simulink model "Ue6_Aufgabe2a"  (R2017a)
settings: Solver=VariableStepAuto  StartTime=0.0  StopTime=50000  RelTol=1e-3
undefined symbols (not defined in the file or in its folder): entity, m, n, showValue, timeStamp
settings Model: Creator=gome  LastModifiedBy=gome

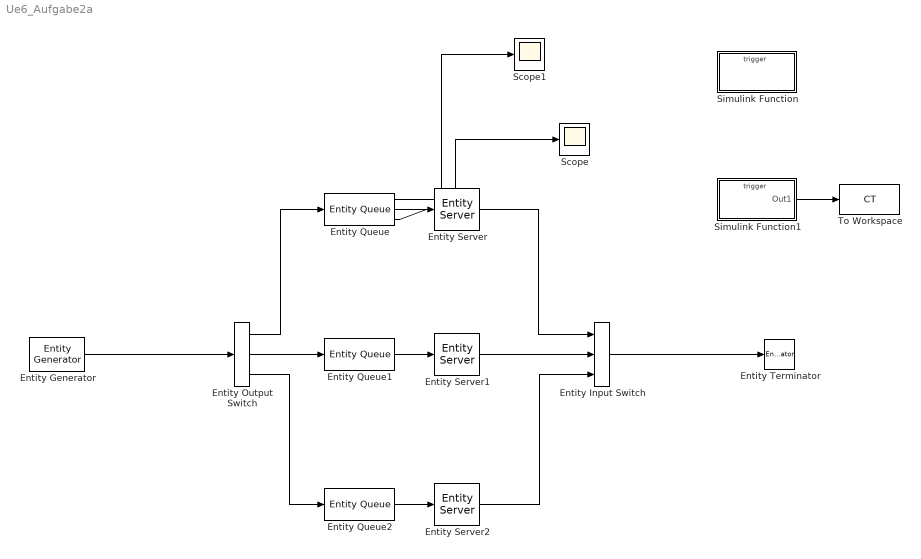
== system Ue6_Aufgabe2a ==
  Entity Input Switch : EntityInputSwitch  InputPortMessageModes=m,m,m  OutputPortMessageModes=m  NumberInputPorts=3
      settings: InputPortMap=u1,u2,u3
  Entity Output Switch : EntityOutputSwitch  InputPortMessageModes=m  OutputPortMessageModes=m,m,m  NumberOutputPorts=3  SwitchingCriterion=Equiprobable  SwitchAttributeName=Attribute1
      settings: OutputPortMap=o0,o1,o2
  Entity Generator : EntityGenerator  OutputPortMessageModes=m  TimeSource=MATLAB action  IntergenerationTimeAction=|  GenerateAction=entity.startTime = timeStamp();  AttributeName=startTime  EntityType=Structured  EntityTypeName=Entity
      | persistent init
      | if isempty(init)
      |     init = 1;
      |     rng(75241);
      | end
      | dt = exprnd(1/2);
  Entity Queue : EntityQueue  InputPortMessageModes=m  OutputPortMessageModes=n,n,m  Capacity=inf  AverageWait=on  AverageQueueLength=on
      settings: OutputPortMap=o2,o3,o5
  Entity Queue1 : EntityQueue  InputPortMessageModes=m  OutputPortMessageModes=m  Capacity=inf
      settings: OutputPortMap=o5
  Entity Queue2 : EntityQueue  InputPortMessageModes=m  OutputPortMessageModes=m  Capacity=inf
      settings: OutputPortMap=o5
  Entity Server : EntityServer  InputPortMessageModes=m  OutputPortMessageModes=m  Capacity=1  ServiceTimeSource=MATLAB action  ServiceTimeAction=|
      | persistent init
      | if isempty(init)
      |     init = 1;
      |     rng(945);
      | end
      | dt = exprnd(1);
  Entity Server1 : EntityServer  InputPortMessageModes=m  OutputPortMessageModes=m  Capacity=1  ServiceTimeSource=MATLAB action  ServiceTimeAction=|
      | persistent init
      | if isempty(init)
      |     init = 1;
      |     rng(1323456);
      | end
      | dt = exprnd(1);
  Entity Server2 : EntityServer  InputPortMessageModes=m  OutputPortMessageModes=m  Capacity=1  ServiceTimeSource=MATLAB action  ServiceTimeAction=|
      | persistent init
      | if isempty(init)
      |     init = 1;
      |     rng(52434);
      | end
      | dt = 0.5+1.5*rand;
  Entity Terminator : EntityTerminator  InputPortMessageModes=m  EntryAction=showValue(timeStamp-entity.startTime);
  Scope : Scope
  Scope1 : Scope
  Simulink Function : Subsystem  TreatAsAtomicUnit=on
  Simulink Function1 : Subsystem  TreatAsAtomicUnit=on
  To Workspace : ToWorkspace  VariableName=CT  SampleTime=-1
  wires:
  Entity Generator/1 -> Entity Output Switch/1
  Entity Output Switch/1 -> Entity Queue/1
  Entity Output Switch/2 -> Entity Queue1/1
  Entity Output Switch/3 -> Entity Queue2/1
  Entity Queue/3 -> Entity Server/1
  Entity Queue1/1 -> Entity Server1/1
  Entity Queue2/1 -> Entity Server2/1
  Entity Server/1 -> Entity Input Switch/1
  Entity Server1/1 -> Entity Input Switch/2
  Entity Server2/1 -> Entity Input Switch/3
  Entity Input Switch/1 -> Entity Terminator/1
  Simulink Function1/1(Out1) -> To Workspace/1
  Entity Queue/1 -> Scope/1
  Entity Queue/2 -> Scope1/1

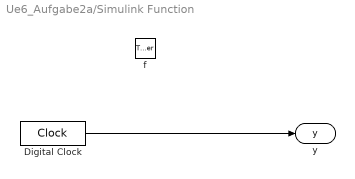
== system Ue6_Aufgabe2a/Simulink Function ==
  f : TriggerPort  TriggerType=function-call  IsSimulinkFunction=on  FunctionName=timeStamp  VariantControl=Variant
  Digital Clock : DigitalClock  SampleTime=-1
  y : ArgOut  DisableCoverage=on  ArgumentName=y
  wires:
  Digital Clock/1 -> y/1

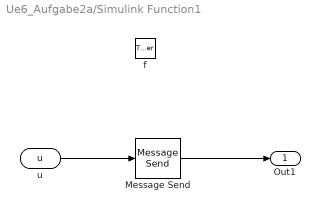
== system Ue6_Aufgabe2a/Simulink Function1 ==
  f : TriggerPort  TriggerType=function-call  IsSimulinkFunction=on  FunctionName=showValue  VariantControl=Variant
  Message Send : MessageSend  OutputPortMessageModes=m
      settings: InputPortMap=u1
  u : ArgIn  DisableCoverage=on  ArgumentName=u
  Out1 : Outport
  wires:
  u/1 -> Message Send/1
  Message Send/1 -> Out1/1
